simulink model "simulation_poursuite"  (Simulink 7.0)
settings: Solver=ode45  StartTime=0.0  StopTime=Temps_Fin  RelTol=1e-6  AbsTol=1e-6
values from neighbouring files (symbols this model uses):
  consigne_bf = 1    [asservissement_2nd_ordre.m]
  pertu_bf = 0    [asservissement_2nd_ordre.m]
  Rd_tf = tf(Rd_i,F)    [mise_en_oeuvre.m]
libraries: cstblocks x5
settings Model: Creator=adminportog  LastModifiedBy=etudiant

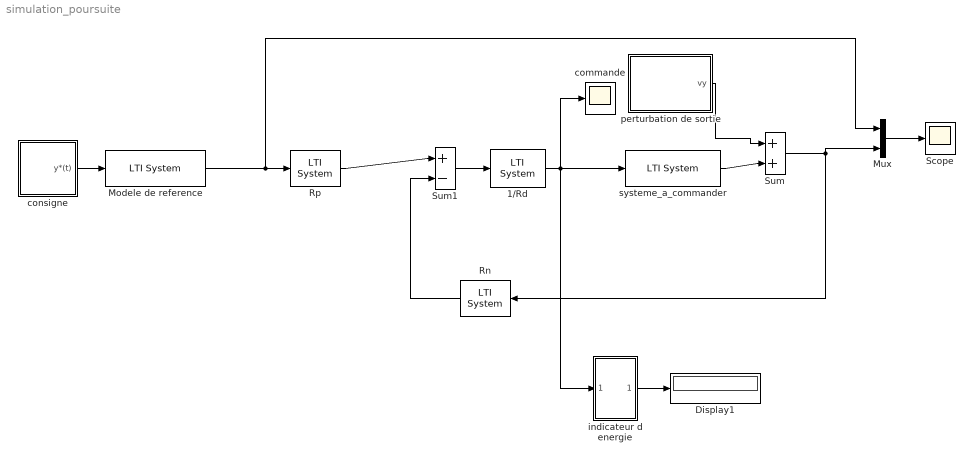
== system simulation_poursuite ==
  1/Rd : cstblocks/LTI System  SystemSampleTime=-1  sys=1/Rd_tf  IC=[]
  Display1 : Display
  Modele de reference : cstblocks/LTI System  SystemSampleTime=-1  sys=modele_reference  IC=[]
  Mux : Mux  Inputs=2
  Rn : cstblocks/LTI System  Orientation=left  SystemSampleTime=-1  sys=Rn_tf  IC=[]
  Rp : cstblocks/LTI System  SystemSampleTime=-1  sys=Rp_tf  IC=[]
  Scope : Scope
      settings: YMin=-1  YMax=1  MaxDataPoints=50000
  Sum : Sum  Inputs=|++  OutDataType=sfix(16)  OutScaling=2^0
  Sum1 : Sum  Inputs=|+-  OutDataType=sfix(16)  OutScaling=2^0
  commande : Scope
      settings: YMin=-300  YMax=300  MaxDataPoints=50000
  consigne : Subsystem
  indicateur d energie : Subsystem
  perturbation de sortie : Subsystem
  systeme_a_commander : cstblocks/LTI System  SystemSampleTime=-1  sys=G1  IC=[]
  wires:
  systeme_a_commander/1 -> Sum/2
  Sum/1 -> Mux/2, Rn/1
  Sum1/1 -> 1/Rd/1
  1/Rd/1 -> systeme_a_commander/1, commande/1, indicateur d energie/1(In1)
  Rn/1 -> Sum1/2
  Rp/1 -> Sum1/1
  Mux/1 -> Scope/1
  Modele de reference/1 -> Rp/1, Mux/1
  consigne/1(y*(t)) -> Modele de reference/1
  perturbation de sortie/1(vy) -> Sum/1
  indicateur d energie/1(Out1) -> Display1/1

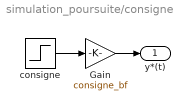
== system simulation_poursuite/consigne ==
  Gain : Gain  Gain=consigne_bf  ParameterDataType=sfix(16)  ParameterScaling=2^0  OutDataType=sfix(16)  OutScaling=2^0
  consigne : Step  Time=0  SampleTime=0
  y*(t) : Outport
  wires:
  consigne/1 -> Gain/1
  Gain/1 -> y*(t)/1

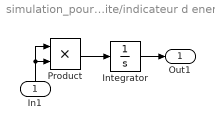
== system simulation_poursuite/indicateur d energie ==
  In1 : Inport  Orientation=up
  Integrator : Integrator
  Product : Product  OutDataType=sfix(16)  OutScaling=2^0  RndMeth=Zero
  Out1 : Outport
  wires:
  Product/1 -> Integrator/1
  In1/1 -> Product/2, Product/1
  Integrator/1 -> Out1/1

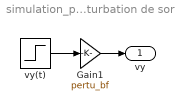
== system simulation_poursuite/perturbation de sortie ==
  Gain1 : Gain  Gain=pertu_bf  ParameterDataType=sfix(16)  ParameterScaling=2^0  OutDataType=sfix(16)  OutScaling=2^0
  vy(t) : Step  Time=5  SampleTime=0
  vy : Outport
  wires:
  vy(t)/1 -> Gain1/1
  Gain1/1 -> vy/1
